simulink model "structured_uncertainty_model"  (R2024b)
settings: Solver=VariableStepAuto  StartTime=0.0  StopTime=10.0  RelTol=1e-3
values from neighbouring files (symbols this model uses):
  K_n = (K_u(1)+K_u(2))/2    [P2.m]
  Wk = (K_u(2)-K_n)/K_n    [P2.m]
  wn_n = (wn_u(1)+wn_u(2))/2    [P2.m]
  Wwn = (wn_u(2)-wn_n)/wn_n    [P2.m]
  Wzeta = (zeta_u(2)-zeta_n)/zeta_n    [P2.m]
  zeta_n = (zeta_u(1)+zeta_u(2))/2    [P2.m]
settings Model: Creator=lucap  LastModifiedBy=lucap

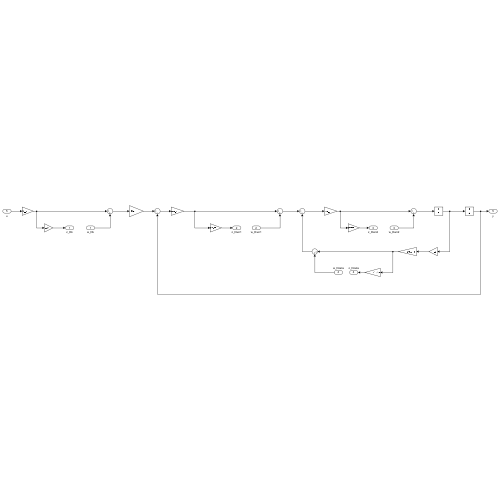
[thumbnail: Simulink's stored preview of the top-level diagram]
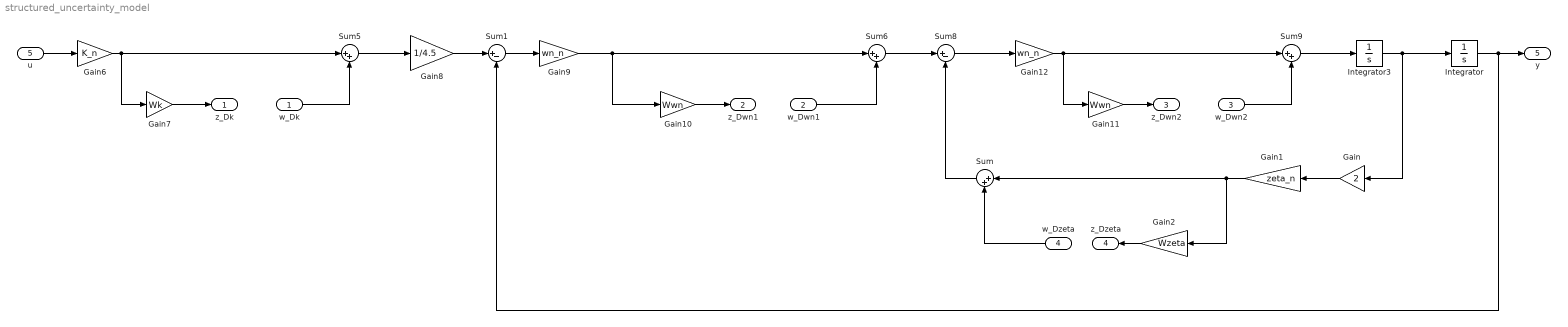
== system structured_uncertainty_model ==
  w_Dk : Inport
  w_Dwn1 : Inport  Port=2
  w_Dwn2 : Inport  Port=3
  w_Dzeta : Inport  Port=4
  u : Inport  Port=5
  Gain : Gain  Gain=2
  Gain1 : Gain  Gain=zeta_n
  Gain10 : Gain  Gain=Wwn
  Gain11 : Gain  Gain=Wwn
  Gain12 : Gain  Gain=wn_n
  Gain2 : Gain  Gain=Wzeta
  Gain6 : Gain  Gain=K_n
  Gain7 : Gain  Gain=Wk
  Gain8 : Gain  Gain=1/4.5
  Gain9 : Gain  Gain=wn_n
  Integrator : Integrator
  Integrator3 : Integrator
  Sum{,5..6,9} (4 alike) : Sum  Inputs=|++
  Sum1 : Sum  Inputs=|+-
  Sum8 : Sum  Inputs=|+-
  z_Dk : Outport
  z_Dwn1 : Outport  Port=2
  z_Dwn2 : Outport  Port=3
  z_Dzeta : Outport  Port=4
  y : Outport  Port=5
  wires:
  Gain6/1 -> Gain7/1, Sum5/1
  Gain7/1 -> z_Dk/1
  w_Dk/1 -> Sum5/2
  Sum5/1 -> Gain8/1
  Gain10/1 -> z_Dwn1/1
  Gain9/1 -> Gain10/1, Sum6/1
  w_Dwn1/1 -> Sum6/2
  w_Dwn2/1 -> Sum9/2
  Gain11/1 -> z_Dwn2/1
  Gain12/1 -> Gain11/1, Sum9/1
  Sum8/1 -> Gain12/1
  Sum9/1 -> Integrator3/1
  Integrator3/1 -> Gain/1, Integrator/1
  Gain/1 -> Gain1/1
  Gain1/1 -> Sum/1, Gain2/1
  Gain2/1 -> z_Dzeta/1
  w_Dzeta/1 -> Sum/2
  Sum/1 -> Sum8/2
  u/1 -> Gain6/1
  Integrator/1 -> Sum1/2, y/1
  Sum6/1 -> Sum8/1
  Sum1/1 -> Gain9/1
  Gain8/1 -> Sum1/1
